simulink model "Controller"  (R2018b)
settings: configuration reference "control_config" (kept outside this file)
values from neighbouring files (symbols this model uses):
  CONTROL_EXPORT = Simulink.Parameter(CONTROL_EXPORT_VALUE)    [base_controller_var.m]    (also in pid_controller_var.m)
  CONTROL_PARAM = Simulink.Parameter(CONTROL_PARAM_VALUE)    [base_controller_var.m]    (also in pid_controller_var.m)
undefined symbols (not defined in the file or in its folder): actuator_cmd, CONTROL_CONST, DiscIntNeverNeededParam, timestamp
libraries: simulink x4, Filter x2, Quaternion x1, Rotation x1
settings Model: Creator=zouji  LastModifiedBy=zouji
settings ConfigSetRef: SourceLocation=Base Workspace

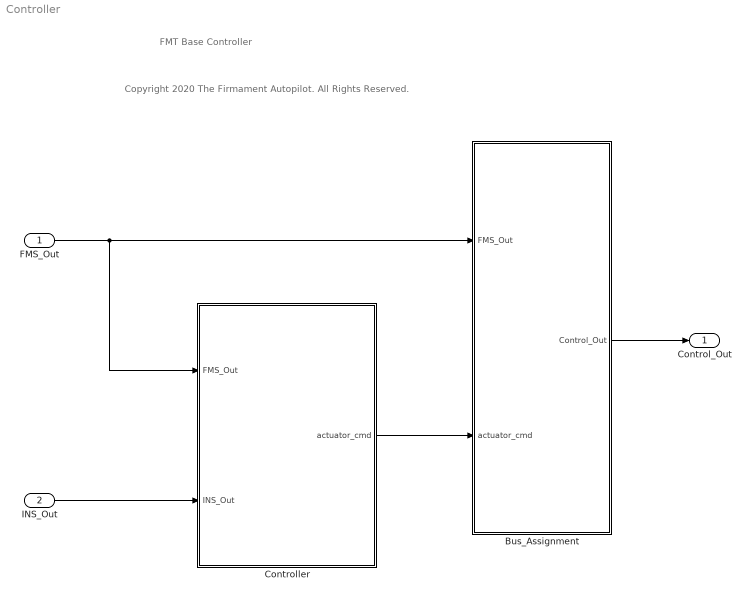
== system Controller ==
  note: Copyright 2020 The Firmament Autopilot. All Rights Reserved.
  note: FMT Base Controller
  FMS_Out : Inport  OutDataTypeStr=Bus: FMS_Out_Bus
  INS_Out : Inport  Port=2  OutDataTypeStr=Bus: INS_Out_Bus
  Bus_Assignment : Subsystem
  Controller : Subsystem
  Control_Out : Outport  OutDataTypeStr=Bus: Control_Out_Bus
  wires:
  FMS_Out/1 -> Controller/1(FMS_Out), Bus_Assignment/1(FMS_Out)
  INS_Out/1 -> Controller/2(INS_Out)
  Controller/1(actuator_cmd) -> Bus_Assignment/2(actuator_cmd)
  Bus_Assignment/1(Control_Out) -> Control_Out/1

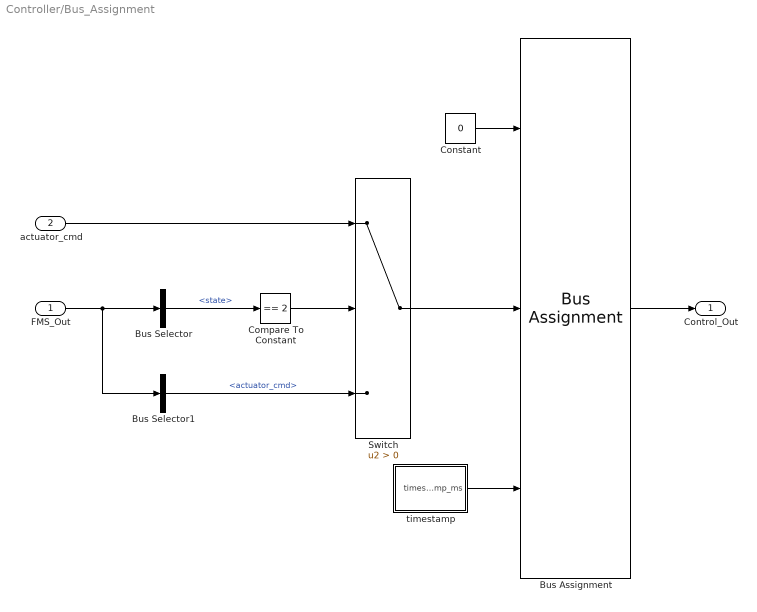
== system Controller/Bus_Assignment ==
  FMS_Out : Inport
  actuator_cmd : Inport  Port=2
  Bus Assignment : BusAssignment  AssignedSignals=actuator_cmd,timestamp
  Bus Selector : BusSelector  OutputSignals=state
  Bus Selector1 : BusSelector  OutputSignals=actuator_cmd
  Compare To Constant : simulink/Logic and Bit Operations/Compare To Constant  relop===  const=2  OutDataTypeStr=boolean
  Constant : Constant  Value=0  OutDataTypeStr=Bus: Control_Out_Bus
  Switch : Switch  Criteria=u2 > Threshold
  timestamp : Subsystem  mask{sample_time=CONTROL_EXPORT.period}
      mask prompts: sample_time "sample time (ms)"
  Control_Out : Outport
  wires:
  FMS_Out/1 -> Bus Selector1/1, Bus Selector/1
  Bus Selector/1 -> Compare To Constant/1  "<state>"
  Bus Selector1/1 -> Switch/3  "<actuator_cmd>"
  Switch/1 -> Bus Assignment/2
  Compare To Constant/1 -> Switch/2
  actuator_cmd/1 -> Switch/1
  Constant/1 -> Bus Assignment/1
  Bus Assignment/1 -> Control_Out/1
  timestamp/1(timestamp_ms) -> Bus Assignment/3

== system Controller/Controller ==
  FMS_Out : Inport
  INS_Out : Inport  Port=2
  Horizontal_Control : Subsystem
  Static_Control_Allocation : Subsystem
  Vertical_Control : Subsystem
  actuator_cmd : Outport
  wires:
  FMS_Out/1 -> Vertical_Control/1(FMS_Out), Horizontal_Control/1(FMS_Out), Static_Control_Allocation/1(FMS_Out)
  INS_Out/1 -> Horizontal_Control/2(INS_Out), Vertical_Control/2(INS_Out)
  Horizontal_Control/1(torque_cmd_normalized) -> Static_Control_Allocation/2(torque_cmd_normalized)
  Vertical_Control/1(thrust_cmd_normalized) -> Static_Control_Allocation/3(thrust_cmd_normalized)
  Static_Control_Allocation/1(actuator_cmd) -> actuator_cmd/1

== system Controller/Bus_Assignment/timestamp ==
  Constant : Constant  Value=sample_time
  Data Type Conversion : DataTypeConversion  OutDataTypeStr=uint32
  Discrete-Time Integrator : DiscreteIntegrator  IntegratorMethod=Accumulation: Forward Euler  SampleTime=-1  ICPrevOutput=DiscIntNeverNeededParam  ICPrevScaledInput=DiscIntNeverNeededParam
  timestamp_ms : Outport
  wires:
  Discrete-Time Integrator/1 -> Data Type Conversion/1
  Constant/1 -> Discrete-Time Integrator/1
  Data Type Conversion/1 -> timestamp_ms/1

== system Controller/Controller/Horizontal_Control ==
  FMS_Out : Inport
  INS_Out : Inport  Port=2
  Attitude_Controller : Subsystem
  Velocity_Controller : Subsystem
  torque_cmd_normalized : Outport
  wires:
  Attitude_Controller/1(torque_cmd_normalized) -> torque_cmd_normalized/1
  FMS_Out/1 -> Attitude_Controller/2(FMS_Out), Velocity_Controller/1(FMS_Out)
  INS_Out/1 -> Velocity_Controller/2(INS_Out), Attitude_Controller/3(INS_Out)
  Velocity_Controller/1(att_cmd_rad) -> Attitude_Controller/1(att_cmd_rad)

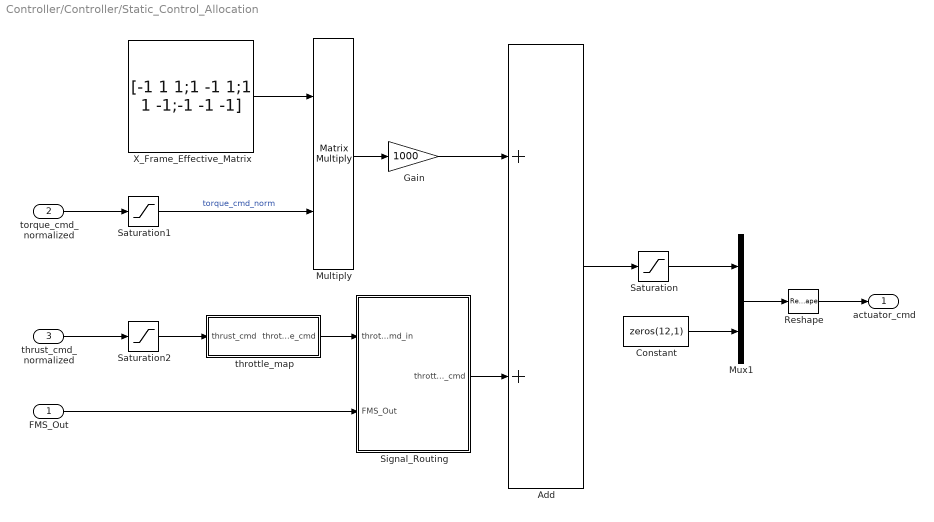
== system Controller/Controller/Static_Control_Allocation ==
  FMS_Out : Inport
  torque_cmd_normalized : Inport  Port=2
  thrust_cmd_normalized : Inport  Port=3
  Add : Sum  OutDataTypeStr=uint16
  Constant : Constant  Value=zeros(12,1)  VectorParams1D=off  OutDataTypeStr=uint16
  Gain : Gain  Gain=1000  OutDataTypeStr=uint16
  Multiply : Product  Multiplication=Matrix(*)  OutDataTypeStr=Inherit: Same as first input
  Mux1 : Mux  Inputs=2
  Reshape : Reshape  OutputDimensionality=Customize  OutputDimensions=[16,1]
  Saturation : Saturate  UpperLimit=2000  LowerLimit=1100
  Saturation1 : Saturate  UpperLimit=1  LowerLimit=-1
  Saturation2 : Saturate  UpperLimit=1  LowerLimit=-1
  Signal_Routing : Subsystem
  X_Frame_Effective_Matrix : Constant  Value=[-1 1 1;1 -1 1;1 1 -1;-1 -1 -1]  OutDataTypeStr=single
  throttle_map : Subsystem
  actuator_cmd : Outport
  wires:
  Multiply/1 -> Gain/1
  X_Frame_Effective_Matrix/1 -> Multiply/1
  torque_cmd_normalized/1 -> Saturation1/1
  Gain/1 -> Add/1
  thrust_cmd_normalized/1 -> Saturation2/1
  Add/1 -> Saturation/1
  Reshape/1 -> actuator_cmd/1
  Mux1/1 -> Reshape/1
  Saturation/1 -> Mux1/1
  Constant/1 -> Mux1/2
  Saturation1/1 -> Multiply/2  "torque_cmd_norm"
  throttle_map/1(throttle_cmd) -> Signal_Routing/1(throttle_cmd_in)
  Signal_Routing/1(throttle_cmd) -> Add/2
  FMS_Out/1 -> Signal_Routing/2(FMS_Out)
  Saturation2/1 -> throttle_map/1(thrust_cmd)

== system Controller/Controller/Vertical_Control ==
  FMS_Out : Inport
  INS_Out : Inport  Port=2
  Veloxity_Z_Controller : Subsystem
  thrust_cmd_normalized : Outport
  wires:
  INS_Out/1 -> Veloxity_Z_Controller/2(INS_Out)
  FMS_Out/1 -> Veloxity_Z_Controller/1(FMS_Out)
  Veloxity_Z_Controller/1(thrust_cmd) -> thrust_cmd_normalized/1

== system Controller/Controller/Horizontal_Control/Attitude_Controller ==
  att_cmd_rad : Inport
  FMS_Out : Inport  Port=2
  INS_Out : Inport  Port=3
  Inner_Loop : Subsystem
  Outter_Loop : Subsystem
  torque_cmd_normalized : Outport
  wires:
  INS_Out/1 -> Inner_Loop/2(INS_Out), Outter_Loop/2(INS_Out)
  FMS_Out/1 -> Outter_Loop/3(FMS_Out), Inner_Loop/3(FMS_Out)
  att_cmd_rad/1 -> Outter_Loop/1(att_cmd_rad)
  Outter_Loop/1(euler_rate_cmd_radPs) -> Inner_Loop/1(euler_rate_cmd_radPs)
  Inner_Loop/1(torque_cmd_normalized) -> torque_cmd_normalized/1

== system Controller/Controller/Horizontal_Control/Velocity_Controller ==
  FMS_Out : Inport
  INS_Out : Inport  Port=2
  Bus Selector : BusSelector  OutputSignals=reset
  Conversion : Subsystem
  Error : Subsystem
  PID_Controller : Subsystem
  Saturation : Saturate  UpperLimit=CONTROL_PARAM.ROLL_PITCH_CMD_LIM  LowerLimit=-CONTROL_PARAM.ROLL_PITCH_CMD_LIM
  att_cmd_rad : Outport
  wires:
  FMS_Out/1 -> Error/2(FMS_Out), Bus Selector/1
  PID_Controller/1(accel_cmd_C) -> Conversion/1(accel_cmd_C)  "accel_cmd_C_mPs2"
  INS_Out/1 -> Error/1(INS_Out)
  Error/1(uv_err_C_mPs) -> PID_Controller/1(uv_err_C_mPs)
  Conversion/1(att_cmd_rad) -> Saturation/1
  Saturation/1 -> att_cmd_rad/1
  Bus Selector/1 -> PID_Controller/2(reset)  "<reset>"

== system Controller/Controller/Static_Control_Allocation/Signal_Routing ==
  note: mode:
      | 0: Unknown
      | 1: Mission
      | 2: Position
      | 3: Altitude Hold
      | 4: Manual Mode
      | 5: Acro Mode
  throttle_cmd_in : Inport
  FMS_Out : Inport  Port=2
  Bus Selector1 : BusSelector  OutputSignals=throttle_cmd,mode
  Compare To Constant : simulink/Logic and Bit Operations/Compare To Constant  relop=>=  const=4  OutDataTypeStr=boolean
  Switch : Switch  Criteria=u2 > Threshold
  throttle_cmd : Outport
  wires:
  Compare To Constant/1 -> Switch/2
  FMS_Out/1 -> Bus Selector1/1
  Bus Selector1/1 -> Switch/1  "<throttle_cmd>"
  Bus Selector1/2 -> Compare To Constant/1  "<mode>"
  Switch/1 -> throttle_cmd/1  "throttle_cmd"
  throttle_cmd_in/1 -> Switch/3

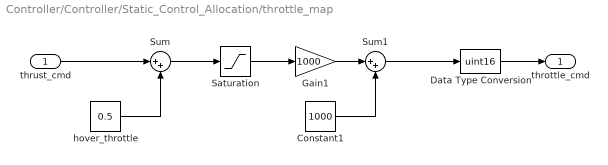
== system Controller/Controller/Static_Control_Allocation/throttle_map ==
  thrust_cmd : Inport
  Constant1 : Constant  Value=1000  OutDataTypeStr=uint32
  Data Type Conversion : DataTypeConversion  OutDataTypeStr=uint16
  Gain1 : Gain  Gain=1000  OutDataTypeStr=uint32
  Saturation : Saturate  UpperLimit=1  LowerLimit=0
  Sum : Sum  Inputs=|++
  Sum1 : Sum  Inputs=|++
  hover_throttle : Constant  Value=0.5  OutDataTypeStr=Inherit: Inherit via back propagation
  throttle_cmd : Outport
  wires:
  thrust_cmd/1 -> Sum/1
  Sum/1 -> Saturation/1
  hover_throttle/1 -> Sum/2
  Gain1/1 -> Sum1/1
  Constant1/1 -> Sum1/2
  Data Type Conversion/1 -> throttle_cmd/1
  Saturation/1 -> Gain1/1
  Sum1/1 -> Data Type Conversion/1

== system Controller/Controller/Vertical_Control/Veloxity_Z_Controller ==
  note: Leave some margin
      | for att control
  FMS_Out : Inport
  INS_Out : Inport  Port=2
  Bus Selector : BusSelector  OutputSignals=reset
  Error : Subsystem
  PID_Controller : Subsystem
  Saturation : Saturate  UpperLimit=0.35  LowerLimit=-0.35
  thrust_cmd : Outport
  wires:
  Bus Selector/1 -> PID_Controller/2(reset)  "<reset>"
  FMS_Out/1 -> Bus Selector/1, Error/1(FMS_Out)
  INS_Out/1 -> PID_Controller/3(INS_Out), Error/2(INS_Out)
  PID_Controller/1(thrust_cmd) -> Saturation/1
  Error/1(h_err_mPs) -> PID_Controller/1(h_err_mPs)
  Saturation/1 -> thrust_cmd/1

== system Controller/Controller/Horizontal_Control/Attitude_Controller/Inner_Loop ==
  euler_rate_cmd_radPs : Inport
  INS_Out : Inport  Port=2
  FMS_Out : Inport  Port=3
  Bus Selector : BusSelector  OutputSignals=reset
  Conversion : Subsystem
  Rate_Controller : Subsystem
  Signal_Routing : Subsystem
  torque_cmd_normalized : Outport
  wires:
  euler_rate_cmd_radPs/1 -> Conversion/2(euler_rate_cmd)
  Signal_Routing/1(out) -> Rate_Controller/1(rate_cmd_radPs)
  Rate_Controller/1(torque_cmd) -> torque_cmd_normalized/1
  Bus Selector/1 -> Rate_Controller/3(reset)  "<reset>"
  INS_Out/1 -> Conversion/3(INS_Out), Rate_Controller/2(INS_Out)
  FMS_Out/1 -> Conversion/1(FMS_Out), Bus Selector/1, Signal_Routing/1(FMS_Out)
  Conversion/1(rate_cmd) -> Signal_Routing/2(rate_cmd_radPs)

== system Controller/Controller/Horizontal_Control/Attitude_Controller/Outter_Loop ==
  att_cmd_rad : Inport
  INS_Out : Inport  Port=2
  FMS_Out : Inport  Port=3
  Attitude_Controller : Subsystem
  Signal_Routing : Subsystem
  euler_rate_cmd_radPs : Outport
  wires:
  Signal_Routing/1(out) -> Attitude_Controller/1(att_cmd_rad)
  FMS_Out/1 -> Signal_Routing/2(FMS_Out)
  INS_Out/1 -> Attitude_Controller/2(INS_Out)
  Attitude_Controller/1(euler_rate_cmd_radPs) -> euler_rate_cmd_radPs/1
  att_cmd_rad/1 -> Signal_Routing/1(att_cmd_rad)

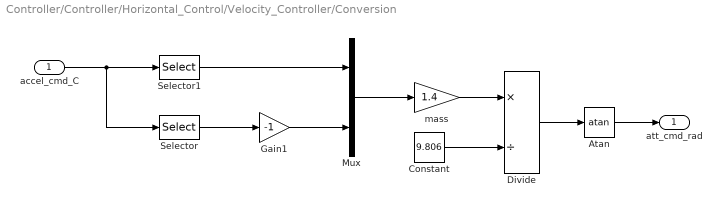
== system Controller/Controller/Horizontal_Control/Velocity_Controller/Conversion ==
  accel_cmd_C : Inport
  Atan : Trigonometry  Operator=atan
  Constant : Constant  Value=9.806  OutDataTypeStr=single
  Divide : Product  Inputs=*/
  Gain1 : Gain  Gain=-1
  Mux : Mux  Inputs=2
  Selector : Selector  InputPortWidth=2  IndexOptions=Index vector (dialog)  Indices=1  OutputSizes=1
  Selector1 : Selector  InputPortWidth=2  IndexOptions=Index vector (dialog)  Indices=2  OutputSizes=1
  mass : Gain  Gain=1.4
  att_cmd_rad : Outport
  wires:
  Mux/1 -> mass/1
  mass/1 -> Divide/1
  Atan/1 -> att_cmd_rad/1
  Constant/1 -> Divide/2
  Divide/1 -> Atan/1
  Selector/1 -> Gain1/1
  Selector1/1 -> Mux/1
  accel_cmd_C/1 -> Selector/1, Selector1/1
  Gain1/1 -> Mux/2

== system Controller/Controller/Horizontal_Control/Velocity_Controller/Error ==
  INS_Out : Inport
  FMS_Out : Inport  Port=2
  Bus Selector : BusSelector  OutputSignals=u_cmd,v_cmd
  Mux : Mux  Inputs=2
  Subsystem : Subsystem
  Sum : Sum  Inputs=|+-
  uv_err_C_mPs : Outport
  wires:
  Sum/1 -> uv_err_C_mPs/1
  FMS_Out/1 -> Bus Selector/1
  INS_Out/1 -> Subsystem/1(INS_Out)
  Bus Selector/1 -> Mux/1  "<u_cmd>"
  Bus Selector/2 -> Mux/2  "<v_cmd>"
  Mux/1 -> Sum/1
  Subsystem/1(uv_C) -> Sum/2  "uv_C_mPs"

== system Controller/Controller/Horizontal_Control/Velocity_Controller/PID_Controller ==
  uv_err_C_mPs : Inport
  reset : Inport  Port=2
  Add : Sum  Inputs=+++
  D_Control : Subsystem  mask{kd=CONTROL_PARAM.VEL_XY_D, max_d=CONTROL_PARAM.VEL_XY_D_MAX, min_d=CONTROL_PARAM.VEL_XY_D_MIN}
  I_Control : Subsystem  mask{ki=CONTROL_PARAM.VEL_XY_I, max_i=CONTROL_PARAM.VEL_XY_I_MAX, min_i=CONTROL_PARAM.VEL_XY_I_MIN}
  P_Control : Subsystem  mask{kp=CONTROL_PARAM.VEL_XY_P}
  accel_cmd_C : Outport
  wires:
  uv_err_C_mPs/1 -> P_Control/1(err), I_Control/1(err), D_Control/1(err)
  reset/1 -> I_Control/2(reset), D_Control/2(reset)
  P_Control/1(p_out) -> Add/1
  I_Control/1(i_out) -> Add/2
  D_Control/1(d_out) -> Add/3
  Add/1 -> accel_cmd_C/1

== system Controller/Controller/Vertical_Control/Veloxity_Z_Controller/Error ==
  FMS_Out : Inport
  INS_Out : Inport  Port=2
  Bus Selector : BusSelector  OutputSignals=w_cmd
  Bus Selector1 : BusSelector  OutputSignals=vd
  Gain : Gain  Gain=-1  OutDataTypeStr=Inherit: Same as input
  Sum1 : Sum  Inputs=|+-
  h_err_mPs : Outport
  wires:
  Bus Selector/1 -> Sum1/1  "<w_cmd>"
  Bus Selector1/1 -> Sum1/2  "<vd>"
  INS_Out/1 -> Bus Selector1/1
  FMS_Out/1 -> Bus Selector/1
  Sum1/1 -> Gain/1  "w_err_mPs"
  Gain/1 -> h_err_mPs/1

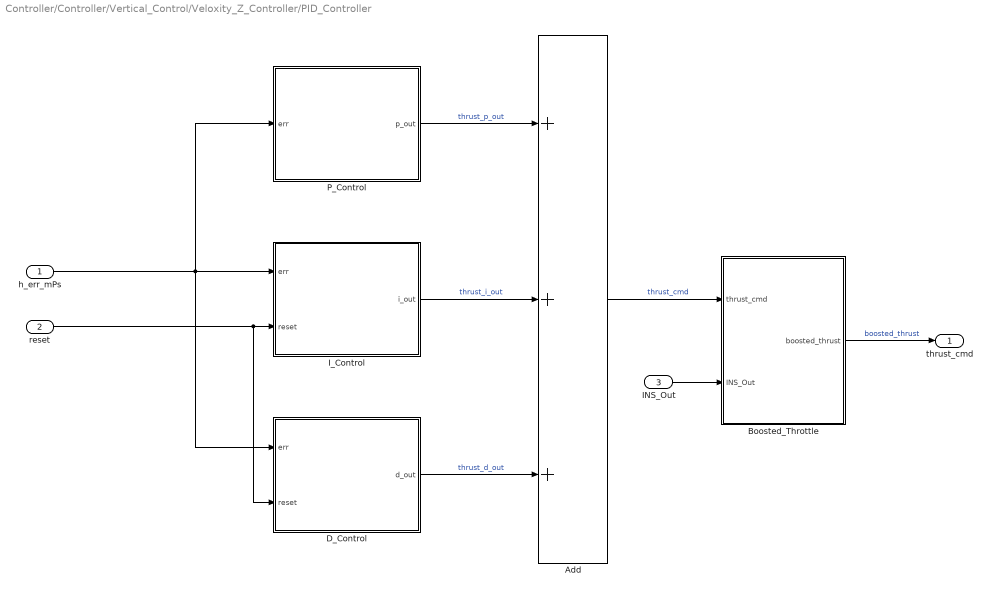
== system Controller/Controller/Vertical_Control/Veloxity_Z_Controller/PID_Controller ==
  h_err_mPs : Inport
  reset : Inport  Port=2
  INS_Out : Inport  Port=3
  Add : Sum  Inputs=+++
  Boosted_Throttle : Subsystem
  D_Control : Subsystem  mask{kd=CONTROL_PARAM.VEL_Z_D, max_d=CONTROL_PARAM.VEL_Z_D_MAX, min_d=CONTROL_PARAM.VEL_Z_D_MIN}
  I_Control : Subsystem  mask{ki=CONTROL_PARAM.VEL_Z_I, max_i=CONTROL_PARAM.VEL_Z_I_MAX, min_i=CONTROL_PARAM.VEL_Z_I_MIN}
  P_Control : Subsystem  mask{kp=CONTROL_PARAM.VEL_Z_P}
  thrust_cmd : Outport
  wires:
  h_err_mPs/1 -> P_Control/1(err), I_Control/1(err), D_Control/1(err)
  reset/1 -> I_Control/2(reset), D_Control/2(reset)
  P_Control/1(p_out) -> Add/1  "thrust_p_out"
  I_Control/1(i_out) -> Add/2  "thrust_i_out"
  D_Control/1(d_out) -> Add/3  "thrust_d_out"
  Add/1 -> Boosted_Throttle/1(thrust_cmd)  "thrust_cmd"
  Boosted_Throttle/1(boosted_thrust) -> thrust_cmd/1  "boosted_thrust"
  INS_Out/1 -> Boosted_Throttle/2(INS_Out)

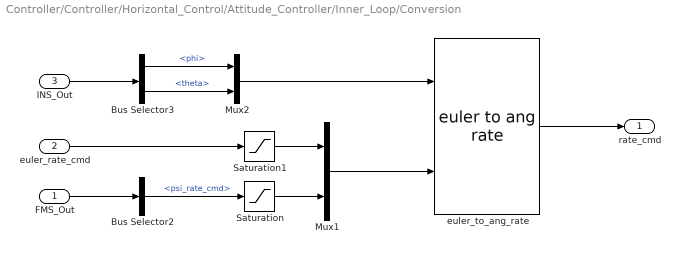
== system Controller/Controller/Horizontal_Control/Attitude_Controller/Inner_Loop/Conversion ==
  FMS_Out : Inport
  euler_rate_cmd : Inport  Port=2
  INS_Out : Inport  Port=3
  Bus Selector2 : BusSelector  OutputSignals=psi_rate_cmd
  Bus Selector3 : BusSelector  OutputSignals=phi,theta
  Mux1 : Mux  Inputs=2
  Mux2 : Mux  Inputs=2
  Saturation : Saturate  UpperLimit=CONTROL_PARAM.R_CMD_LIM  LowerLimit=-CONTROL_PARAM.R_CMD_LIM
  Saturation1 : Saturate  UpperLimit=CONTROL_PARAM.P_Q_CMD_LIM  LowerLimit=-CONTROL_PARAM.P_Q_CMD_LIM
  euler_to_ang_rate : Quaternion/euler to ang rate  SystemSampleTime=-1
  rate_cmd : Outport
  wires:
  Bus Selector3/1 -> Mux2/1  "<phi>"
  Mux2/1 -> euler_to_ang_rate/1
  Bus Selector3/2 -> Mux2/2  "<theta>"
  euler_rate_cmd/1 -> Saturation1/1
  Bus Selector2/1 -> Saturation/1  "<psi_rate_cmd>"
  Mux1/1 -> euler_to_ang_rate/2
  FMS_Out/1 -> Bus Selector2/1
  INS_Out/1 -> Bus Selector3/1
  euler_to_ang_rate/1 -> rate_cmd/1
  Saturation/1 -> Mux1/2
  Saturation1/1 -> Mux1/1

== system Controller/Controller/Horizontal_Control/Attitude_Controller/Inner_Loop/Rate_Controller ==
  rate_cmd_radPs : Inport
  INS_Out : Inport  Port=2
  reset : Inport  Port=3
  Error : Subsystem
  PID_Controller : Subsystem
  torque_cmd : Outport
  wires:
  INS_Out/1 -> Error/2(INS_Out)
  Error/1(rate_err_radPs) -> PID_Controller/1(rate_err_radPs)
  rate_cmd_radPs/1 -> Error/1(rate_sp)
  reset/1 -> PID_Controller/2(reset)
  PID_Controller/1(torque_cmd) -> torque_cmd/1  "torque_cmd"

== system Controller/Controller/Horizontal_Control/Attitude_Controller/Inner_Loop/Signal_Routing ==
  note: mode:
      | 0: Unknown
      | 1: Mission
      | 2: Stablize
      | 3: Altitude Hold
      | 4: Attitude Mode
      | 5: Acro Mode
  FMS_Out : Inport
  rate_cmd_radPs : Inport  Port=2
  Bus Selector : BusSelector  OutputSignals=mode
  Bus Selector1 : BusSelector  OutputSignals=p_cmd,q_cmd,r_cmd
  Compare To Constant : simulink/Logic and Bit Operations/Compare To Constant  relop===  const=5  OutDataTypeStr=boolean
  Mux : Mux  Inputs=3
  Switch : Switch  Criteria=u2 > Threshold
  out : Outport
  wires:
  FMS_Out/1 -> Bus Selector1/1, Bus Selector/1
  Switch/1 -> out/1
  Bus Selector/1 -> Compare To Constant/1  "<mode>"
  Compare To Constant/1 -> Switch/2
  Bus Selector1/1 -> Mux/1  "<p_cmd>"
  Bus Selector1/2 -> Mux/2  "<q_cmd>"
  Bus Selector1/3 -> Mux/3  "<r_cmd>"
  Mux/1 -> Switch/1
  rate_cmd_radPs/1 -> Switch/3

== system Controller/Controller/Horizontal_Control/Attitude_Controller/Outter_Loop/Attitude_Controller ==
  att_cmd_rad : Inport
  INS_Out : Inport  Port=2
  Error : Subsystem
  Non_Linear_P_Controller : Subsystem
  euler_rate_cmd_radPs : Outport
  wires:
  INS_Out/1 -> Error/2(INS_Out)
  Error/1(att_err_rad) -> Non_Linear_P_Controller/1(att_err)
  Non_Linear_P_Controller/1(euler_rate_cmd_radPs) -> euler_rate_cmd_radPs/1
  att_cmd_rad/1 -> Error/1(att_cmd)

== system Controller/Controller/Horizontal_Control/Attitude_Controller/Outter_Loop/Signal_Routing ==
  note: mode:
      | 0: Unknown
      | 1: Mission
      | 2: Position
      | 3: Altitude Hold
      | 4: Manual Mode
      | 5: Acro Mode
  att_cmd_rad : Inport
  FMS_Out : Inport  Port=2
  Bus Selector : BusSelector  OutputSignals=mode
  Bus Selector1 : BusSelector  OutputSignals=phi_cmd,theta_cmd
  Compare To Constant : simulink/Logic and Bit Operations/Compare To Constant  relop=>=  const=3  OutDataTypeStr=boolean
  Mux : Mux  Inputs=2
  Switch : Switch  Criteria=u2 > Threshold
  out : Outport
  wires:
  Compare To Constant/1 -> Switch/2
  Bus Selector1/2 -> Mux/2  "<theta_cmd>"
  Bus Selector1/1 -> Mux/1  "<phi_cmd>"
  att_cmd_rad/1 -> Switch/3
  Bus Selector/1 -> Compare To Constant/1  "<mode>"
  FMS_Out/1 -> Bus Selector1/1, Bus Selector/1
  Mux/1 -> Switch/1
  Switch/1 -> out/1

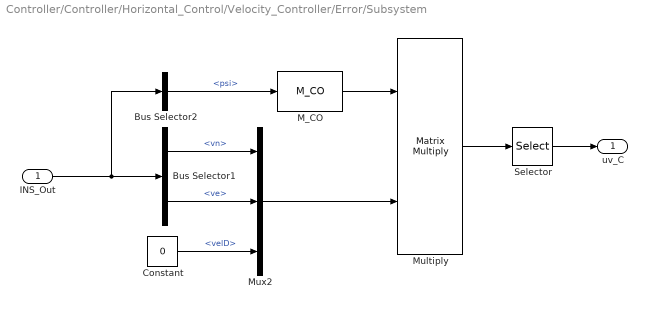
== system Controller/Controller/Horizontal_Control/Velocity_Controller/Error/Subsystem ==
  INS_Out : Inport
  Bus Selector1 : BusSelector  OutputSignals=vn,ve
  Bus Selector2 : BusSelector  OutputSignals=psi
  Constant : Constant  Value=0  OutDataTypeStr=single
  M_CO : Rotation/M_CO  SystemSampleTime=-1
  Multiply : Product  Multiplication=Matrix(*)
  Mux2 : Mux  Inputs=3
  Selector : Selector  InputPortWidth=3  IndexOptions=Index vector (dialog)  Indices=[1 2]  OutputSizes=1
  uv_C : Outport
  wires:
  M_CO/1 -> Multiply/1
  Bus Selector2/1 -> M_CO/1  "<psi>"
  Constant/1 -> Mux2/3  "<velD>"
  Mux2/1 -> Multiply/2
  Bus Selector1/2 -> Mux2/2  "<ve>"
  Bus Selector1/1 -> Mux2/1  "<vn>"
  INS_Out/1 -> Bus Selector2/1, Bus Selector1/1
  Multiply/1 -> Selector/1
  Selector/1 -> uv_C/1

== system Controller/Controller/Horizontal_Control/Velocity_Controller/PID_Controller/D_Control ==
  err : Inport
  reset : Inport  Port=2
  DT1_Filter : Subsystem  mask{T_filter=0.1}
      mask prompts: T_filter "Time constant [s]"
      mask Display: fprintf('T = %.3f', T_filter)
  Multiply : Product  OutDataTypeStr=Inherit: Same as first input
  Saturation : Saturate  UpperLimit=max_d  LowerLimit=min_d
  kd : Constant  Value=kd  OutDataTypeStr=single
  d_out : Outport
  wires:
  err/1 -> DT1_Filter/1(u)
  kd/1 -> Multiply/1
  Multiply/1 -> Saturation/1
  DT1_Filter/1(y) -> Multiply/2
  Saturation/1 -> d_out/1
  reset/1 -> DT1_Filter/2(reset)

== system Controller/Controller/Horizontal_Control/Velocity_Controller/PID_Controller/I_Control ==
  err : Inport
  reset : Inport  Port=2
  Constant : Constant  Value=0  OutDataTypeStr=single
  Discrete-Time Integrator : DiscreteIntegrator  ExternalReset=level  InitialConditionSource=external  SampleTime=-1  LimitOutput=on  UpperSaturationLimit=max_i  LowerSaturationLimit=min_i  ICPrevOutput=DiscIntNeverNeededParam  ICPrevScaledInput=DiscIntNeverNeededParam
  Multiply : Product  OutDataTypeStr=Inherit: Same as first input
  ki : Constant  Value=ki  OutDataTypeStr=single
  i_out : Outport
  wires:
  err/1 -> Multiply/2
  Multiply/1 -> Discrete-Time Integrator/1
  reset/1 -> Discrete-Time Integrator/2
  Constant/1 -> Discrete-Time Integrator/3
  Discrete-Time Integrator/1 -> i_out/1
  ki/1 -> Multiply/1

== system Controller/Controller/Horizontal_Control/Velocity_Controller/PID_Controller/P_Control ==
  err : Inport
  Multiply : Product  OutDataTypeStr=Inherit: Same as first input
  kp : Constant  Value=kp  OutDataTypeStr=single
  p_out : Outport
  wires:
  err/1 -> Multiply/2
  kp/1 -> Multiply/1
  Multiply/1 -> p_out/1

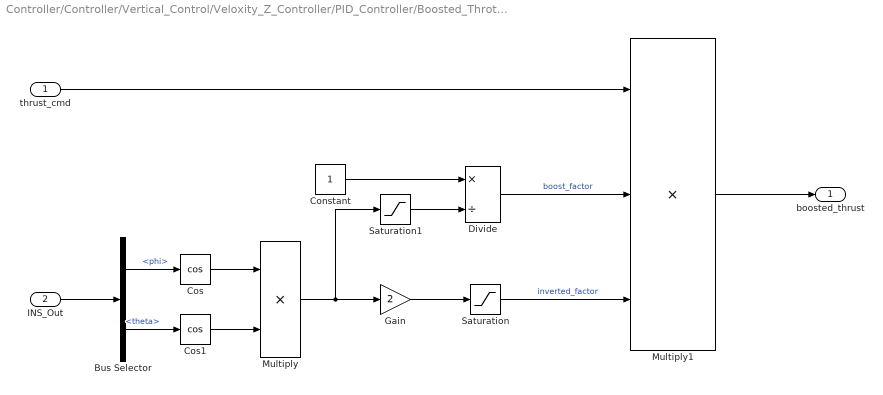
== system Controller/Controller/Vertical_Control/Veloxity_Z_Controller/PID_Controller/Boosted_Throttle ==
  thrust_cmd : Inport
  INS_Out : Inport  Port=2
  Bus Selector : BusSelector  OutputSignals=phi,theta
  Constant : Constant  OutDataTypeStr=single
  Cos : Trigonometry  Operator=cos
  Cos1 : Trigonometry  Operator=cos
  Divide : Product  Inputs=*/
  Gain : Gain  Gain=2
  Multiply : Product
  Multiply1 : Product  Inputs=3
  Saturation : Saturate  UpperLimit=1  LowerLimit=0
  Saturation1 : Saturate  UpperLimit=1  LowerLimit=0.5
  boosted_thrust : Outport
  wires:
  INS_Out/1 -> Bus Selector/1
  Bus Selector/1 -> Cos/1  "<phi>"
  Bus Selector/2 -> Cos1/1  "<theta>"
  Cos/1 -> Multiply/1
  Cos1/1 -> Multiply/2
  Multiply/1 -> Saturation1/1, Gain/1
  Gain/1 -> Saturation/1
  Saturation/1 -> Multiply1/3  "inverted_factor"
  Constant/1 -> Divide/1
  Divide/1 -> Multiply1/2  "boost_factor"
  Saturation1/1 -> Divide/2
  thrust_cmd/1 -> Multiply1/1
  Multiply1/1 -> boosted_thrust/1

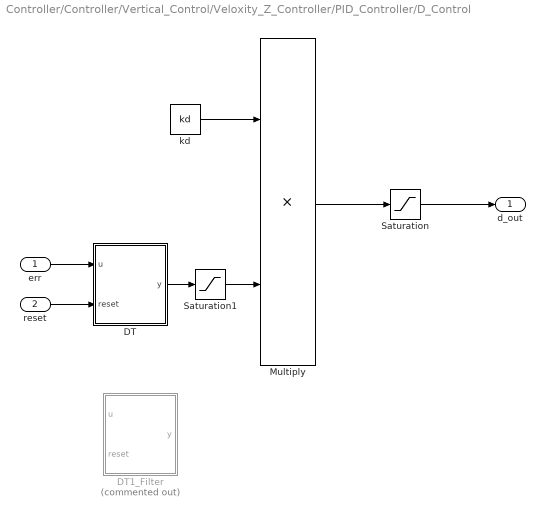
== system Controller/Controller/Vertical_Control/Veloxity_Z_Controller/PID_Controller/D_Control ==
  err : Inport
  reset : Inport  Port=2
  DT : Subsystem  mask{wn=5}
      mask prompts: wn "Cut-off freq (Hz)"
  DT1_Filter : Subsystem  Commented=on  mask{T_filter=0.2}
      mask prompts: T_filter "Time constant [s]"
      mask Display: fprintf('T = %.3f', T_filter)
  Multiply : Product  OutDataTypeStr=Inherit: Same as first input
  Saturation : Saturate  UpperLimit=max_d  LowerLimit=min_d
  Saturation1 : Saturate  UpperLimit=20  LowerLimit=-20
  kd : Constant  Value=kd  OutDataTypeStr=single
  d_out : Outport
  wires:
  err/1 -> DT/1(u)
  kd/1 -> Multiply/1
  Multiply/1 -> Saturation/1
  Saturation/1 -> d_out/1
  reset/1 -> DT/2(reset)
  DT/1(y) -> Saturation1/1
  Saturation1/1 -> Multiply/2

== system Controller/Controller/Vertical_Control/Veloxity_Z_Controller/PID_Controller/I_Control ==
  err : Inport
  reset : Inport  Port=2
  Constant : Constant  Value=0  OutDataTypeStr=single
  Discrete-Time Integrator : DiscreteIntegrator  ExternalReset=level  InitialConditionSource=external  SampleTime=-1  LimitOutput=on  UpperSaturationLimit=max_i  LowerSaturationLimit=min_i  ICPrevOutput=DiscIntNeverNeededParam  ICPrevScaledInput=DiscIntNeverNeededParam
  Multiply : Product  OutDataTypeStr=Inherit: Same as first input
  ki : Constant  Value=ki  OutDataTypeStr=single
  i_out : Outport
  wires:
  err/1 -> Multiply/2
  Multiply/1 -> Discrete-Time Integrator/1
  reset/1 -> Discrete-Time Integrator/2
  Constant/1 -> Discrete-Time Integrator/3
  Discrete-Time Integrator/1 -> i_out/1
  ki/1 -> Multiply/1

== system Controller/Controller/Vertical_Control/Veloxity_Z_Controller/PID_Controller/P_Control ==
  err : Inport
  Multiply : Product  OutDataTypeStr=Inherit: Same as first input
  kp : Constant  Value=kp  OutDataTypeStr=single
  p_out : Outport
  wires:
  err/1 -> Multiply/2
  kp/1 -> Multiply/1
  Multiply/1 -> p_out/1

== system Controller/Controller/Horizontal_Control/Attitude_Controller/Inner_Loop/Rate_Controller/Error ==
  rate_sp : Inport
  INS_Out : Inport  Port=2
  Bus Selector1 : BusSelector  OutputSignals=p,q,r
  Mux1 : Mux  Inputs=3
  PT_Filter : Subsystem  Commented=through  mask{T_filter=0.05}
      mask prompts: T_filter "Time constant [s]"
      mask Display: fprintf('T = %.3f', T_filter)
  Sum : Sum  Inputs=|+-
  rate_err_radPs : Outport
  wires:
  Bus Selector1/2 -> Mux1/2  "<q>"
  Bus Selector1/3 -> Mux1/3  "<r>"
  Bus Selector1/1 -> Mux1/1  "<p>"
  INS_Out/1 -> Bus Selector1/1
  Mux1/1 -> Sum/2  "rate_est_radPs"
  Sum/1 -> PT_Filter/1(u)  "rate_err"
  rate_sp/1 -> Sum/1  "rate_cmd_radPs"
  PT_Filter/1(y) -> rate_err_radPs/1

== system Controller/Controller/Horizontal_Control/Attitude_Controller/Inner_Loop/Rate_Controller/PID_Controller ==
  rate_err_radPs : Inport
  reset : Inport  Port=2
  Add : Sum  Inputs=+++
  D_Control : Subsystem  mask{p_kd=CONTROL_PARAM.ROLL_RATE_D, q_kd=CONTROL_PARAM.PITCH_RATE_D, r_kd=CONTROL_PARAM.YAW_RATE_D, max_d=CONTROL_PARAM.RATE_D_MAX, min_d=CONTROL_PARAM.RATE_D_MIN}
  I_Control : Subsystem  mask{p_ki=CONTROL_PARAM.ROLL_RATE_I, q_ki=CONTROL_PARAM.PITCH_RATE_I, r_ki=CONTROL_PARAM.YAW_RATE_I, max_i=CONTROL_PARAM.RATE_I_MAX, min_i=CONTROL_PARAM.RATE_I_MIN}
  P_Control : Subsystem  mask{p_kp=CONTROL_PARAM.ROLL_RATE_P, q_kp=CONTROL_PARAM.PITCH_RATE_P, r_kp=CONTROL_PARAM.YAW_RATE_P}
  torque_cmd : Outport
  wires:
  rate_err_radPs/1 -> P_Control/1(err), I_Control/1(err), D_Control/1(err)
  P_Control/1(p_out) -> Add/1  "torque_p_out"
  I_Control/1(i_out) -> Add/2  "torque_i_out"
  D_Control/1(d_out) -> Add/3  "torque_d_out"
  reset/1 -> I_Control/2(reset), D_Control/2(reset)
  Add/1 -> torque_cmd/1

== system Controller/Controller/Horizontal_Control/Attitude_Controller/Outter_Loop/Attitude_Controller/Error ==
  att_cmd : Inport
  INS_Out : Inport  Port=2
  Bus Selector1 : BusSelector  OutputSignals=phi,theta
  Mux1 : Mux  Inputs=2
  Sum : Sum  Inputs=|+-
  att_err_rad : Outport
  wires:
  Bus Selector1/2 -> Mux1/2  "<theta>"
  Bus Selector1/1 -> Mux1/1  "<phi>"
  INS_Out/1 -> Bus Selector1/1
  Mux1/1 -> Sum/2  "att_est_rad"
  att_cmd/1 -> Sum/1  "att_cmd_rad"
  Sum/1 -> att_err_rad/1  "att_err_rad"

== system Controller/Controller/Horizontal_Control/Attitude_Controller/Outter_Loop/Attitude_Controller/Non_Linear_P_Controller ==
  note: tanh
  att_err : Inport
  Demux : Demux  Outputs=2
  Gain : Gain  Gain=CONTROL_PARAM.ROLL_P
  Gain1 : Gain  Gain=CONTROL_PARAM.PITCH_P
  Gain2 : Gain  Gain=CONTROL_PARAM.P_Q_CMD_LIM
  Mux : Mux  Inputs=2
  Tanh : Trigonometry  Operator=tanh
  euler_rate_cmd_radPs : Outport
  wires:
  Gain2/1 -> euler_rate_cmd_radPs/1
  Gain1/1 -> Mux/2
  Gain/1 -> Mux/1
  Tanh/1 -> Gain2/1
  Demux/2 -> Gain1/1
  Demux/1 -> Gain/1
  att_err/1 -> Demux/1
  Mux/1 -> Tanh/1

== system Controller/Controller/Horizontal_Control/Velocity_Controller/PID_Controller/D_Control/DT1_Filter ==
  u : Inport
  reset : Inport  Port=2
  Discrete-Time Integrator1 : DiscreteIntegrator  ExternalReset=level  SampleTime=-1  ICPrevOutput=DiscIntNeverNeededParam  ICPrevScaledInput=DiscIntNeverNeededParam
  Sum5 : Sum  Inputs=|+-
  k_pt : Gain  Gain=1/T_filter  OutDataTypeStr=Inherit: Same as input
  y : Outport
  wires:
  u/1 -> Sum5/1
  Sum5/1 -> k_pt/1
  Discrete-Time Integrator1/1 -> Sum5/2
  k_pt/1 -> Discrete-Time Integrator1/1, y/1
  reset/1 -> Discrete-Time Integrator1/2

== system Controller/Controller/Vertical_Control/Veloxity_Z_Controller/PID_Controller/D_Control/DT ==
  u : Inport
  reset : Inport  Port=2
  1/T : Gain  Gain=1/CONTROL_CONST.dt  OutDataTypeStr=Inherit: Same as input
  Alpha_LPF : Filter/Alpha_LPF  wn=wn  dt=CONTROL_CONST.dt
  Delay : Delay  DelayLength=1  InitialConditionSource=Input port  ExternalReset=Level
      settings: InputPortMap=u0,r5,p4
  Sum : Sum  Inputs=|+-
  Switch : Switch  Criteria=u2 > Threshold
  zero : Gain  Gain=0  OutDataTypeStr=Inherit: Same as input
  y : Outport
  wires:
  1/T/1 -> Switch/3
  Sum/1 -> zero/1, 1/T/1
  Alpha_LPF/1 -> Sum/1, Delay/1, Delay/3
  Delay/1 -> Sum/2
  u/1 -> Alpha_LPF/1
  reset/1 -> Switch/2, Delay/2, Alpha_LPF/2
  Switch/1 -> y/1
  zero/1 -> Switch/1

== system Controller/Controller/Vertical_Control/Veloxity_Z_Controller/PID_Controller/D_Control/DT1_Filter ==
  u : Inport
  reset : Inport  Port=2
  Discrete-Time Integrator1 : DiscreteIntegrator  ExternalReset=level  SampleTime=-1  ICPrevOutput=DiscIntNeverNeededParam  ICPrevScaledInput=DiscIntNeverNeededParam
  Sum5 : Sum  Inputs=|+-
  k_pt : Gain  Gain=1/T_filter  OutDataTypeStr=Inherit: Same as input
  y : Outport
  wires:
  u/1 -> Sum5/1
  Sum5/1 -> k_pt/1
  Discrete-Time Integrator1/1 -> Sum5/2
  k_pt/1 -> Discrete-Time Integrator1/1, y/1
  reset/1 -> Discrete-Time Integrator1/2

== system Controller/Controller/Horizontal_Control/Attitude_Controller/Inner_Loop/Rate_Controller/Error/PT_Filter ==
  u : Inport
  Discrete-Time Integrator1 : DiscreteIntegrator  InitialConditionSource=external  SampleTime=-1  OutDataTypeStr=single  ICPrevOutput=DiscIntNeverNeededParam  ICPrevScaledInput=DiscIntNeverNeededParam
  Sum5 : Sum  Inputs=|+-
  k_pt : Gain  Gain=1/T_filter
  y : Outport
  wires:
  k_pt/1 -> Discrete-Time Integrator1/1
  Discrete-Time Integrator1/1 -> Sum5/2, y/1
  Sum5/1 -> k_pt/1
  u/1 -> Sum5/1, Discrete-Time Integrator1/2

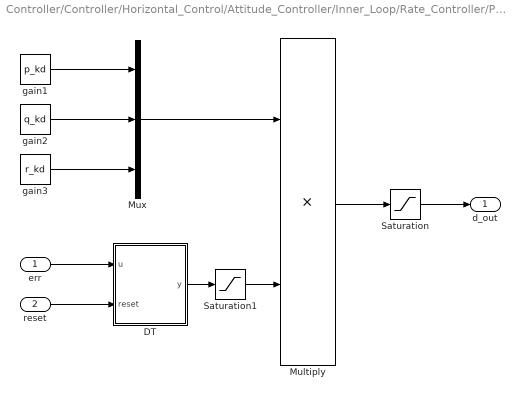
== system Controller/Controller/Horizontal_Control/Attitude_Controller/Inner_Loop/Rate_Controller/PID_Controller/D_Control ==
  err : Inport
  reset : Inport  Port=2
  DT : Subsystem  mask{wn=30}
      mask prompts: wn "Cut-off freq (Hz)"
      mask Display: fprintf('wn = %d Hz', wn)
  Multiply : Product  OutDataTypeStr=Inherit: Same as first input
  Mux : Mux  Inputs=3
  Saturation : Saturate  UpperLimit=max_d  LowerLimit=min_d
  Saturation1 : Saturate  UpperLimit=20  LowerLimit=-20
  gain1 : Constant  Value=p_kd  OutDataTypeStr=single
  gain2 : Constant  Value=q_kd  OutDataTypeStr=single
  gain3 : Constant  Value=r_kd  OutDataTypeStr=single
  d_out : Outport
  wires:
  err/1 -> DT/1(u)
  gain2/1 -> Mux/2
  gain1/1 -> Mux/1
  Multiply/1 -> Saturation/1
  gain3/1 -> Mux/3
  DT/1(y) -> Saturation1/1
  Saturation/1 -> d_out/1
  reset/1 -> DT/2(reset)
  Mux/1 -> Multiply/1
  Saturation1/1 -> Multiply/2

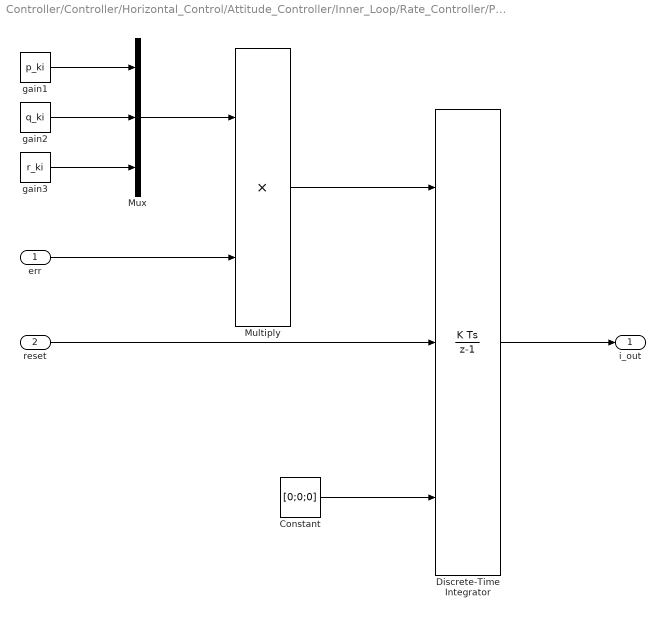
== system Controller/Controller/Horizontal_Control/Attitude_Controller/Inner_Loop/Rate_Controller/PID_Controller/I_Control ==
  err : Inport
  reset : Inport  Port=2
  Constant : Constant  Value=[0;0;0]  OutDataTypeStr=single
  Discrete-Time Integrator : DiscreteIntegrator  ExternalReset=level  InitialConditionSource=external  SampleTime=-1  LimitOutput=on  UpperSaturationLimit=max_i  LowerSaturationLimit=min_i  ICPrevOutput=DiscIntNeverNeededParam  ICPrevScaledInput=DiscIntNeverNeededParam
  Multiply : Product  OutDataTypeStr=Inherit: Same as first input
  Mux : Mux  Inputs=3
  gain1 : Constant  Value=p_ki  OutDataTypeStr=single
  gain2 : Constant  Value=q_ki  OutDataTypeStr=single
  gain3 : Constant  Value=r_ki  OutDataTypeStr=single
  i_out : Outport
  wires:
  err/1 -> Multiply/2
  gain2/1 -> Mux/2
  Mux/1 -> Multiply/1
  gain1/1 -> Mux/1
  gain3/1 -> Mux/3
  Multiply/1 -> Discrete-Time Integrator/1
  reset/1 -> Discrete-Time Integrator/2
  Constant/1 -> Discrete-Time Integrator/3
  Discrete-Time Integrator/1 -> i_out/1

== system Controller/Controller/Horizontal_Control/Attitude_Controller/Inner_Loop/Rate_Controller/PID_Controller/P_Control ==
  err : Inport
  Multiply : Product  OutDataTypeStr=Inherit: Same as first input
  Mux : Mux  Inputs=3
  gain1 : Constant  Value=p_kp  OutDataTypeStr=single
  gain2 : Constant  Value=q_kp  OutDataTypeStr=single
  gain3 : Constant  Value=r_kp  OutDataTypeStr=single
  p_out : Outport
  wires:
  err/1 -> Multiply/2
  gain2/1 -> Mux/2
  Mux/1 -> Multiply/1
  gain1/1 -> Mux/1
  Multiply/1 -> p_out/1
  gain3/1 -> Mux/3

== system Controller/Controller/Horizontal_Control/Attitude_Controller/Inner_Loop/Rate_Controller/PID_Controller/D_Control/DT ==
  u : Inport
  reset : Inport  Port=2
  1/T : Gain  Gain=1/CONTROL_CONST.dt  OutDataTypeStr=Inherit: Same as input
  Alpha_LPF : Filter/Alpha_LPF  wn=wn  dt=CONTROL_CONST.dt
  Delay : Delay  DelayLength=1  InitialConditionSource=Input port  ExternalReset=Level
      settings: InputPortMap=u0,r5,p4
  Sum : Sum  Inputs=|+-
  Switch : Switch  Criteria=u2 > Threshold
  zero : Gain  Gain=0  OutDataTypeStr=Inherit: Same as input
  y : Outport
  wires:
  1/T/1 -> Switch/3
  Sum/1 -> zero/1, 1/T/1
  Alpha_LPF/1 -> Sum/1, Delay/1, Delay/3
  Delay/1 -> Sum/2
  u/1 -> Alpha_LPF/1
  reset/1 -> Switch/2, Delay/2, Alpha_LPF/2
  Switch/1 -> y/1
  zero/1 -> Switch/1
